simulink model "admittance_slx"  (R2020a)
settings: Solver=VariableStepAuto  StartTime=0.0  StopTime=10  MaxStep=0.0005  RelTol=1e-3
settings Model: Creator=AO  LastModifiedBy=jinqiyuan
settings DataIOCC: ReturnWorkspaceOutputs=off

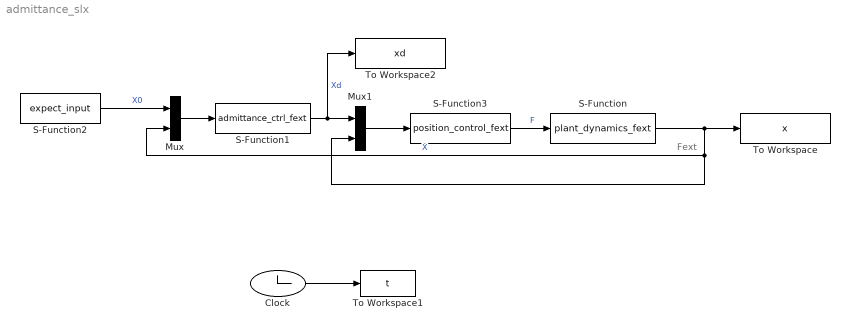
== system admittance_slx ==
  note: Fext
  Clock : Clock
      settings: Decimation=20
  Mux : Mux  Inputs=2
  Mux1 : Mux  Inputs=2
  S-Function : S-Function  FunctionName=plant_dynamics_fext  SFunctionDeploymentMode=off  EnableBusSupport=off
  S-Function1 : S-Function  FunctionName=admittance_ctrl_fext  SFunctionDeploymentMode=off  EnableBusSupport=off
  S-Function2 : S-Function  FunctionName=expect_input  SFunctionDeploymentMode=off  EnableBusSupport=off
  S-Function3 : S-Function  FunctionName=position_control_fext  SFunctionDeploymentMode=off  EnableBusSupport=off
  To Workspace : ToWorkspace  VariableName=x  SampleTime=-1
  To Workspace1 : ToWorkspace  VariableName=t  SampleTime=-1
  To Workspace2 : ToWorkspace  VariableName=xd  SampleTime=-1
  wires:
  Mux/1 -> S-Function1/1
  Clock/1 -> To Workspace1/1
  S-Function/1 -> Mux/2, Mux1/2, To Workspace/1  "X"
  Mux1/1 -> S-Function3/1
  S-Function1/1 -> To Workspace2/1, Mux1/1  "Xd"
  S-Function2/1 -> Mux/1  "X0"
  S-Function3/1 -> S-Function/1  "F"
